simulink model "AccelerationValidation"  (R2022b)
settings: Solver=VariableStepAuto  StartTime=0.0  StopTime=10.0  RelTol=1e-3
(part 1 of 2)
settings Model: Creator=DELL  LastModifiedBy=DELL

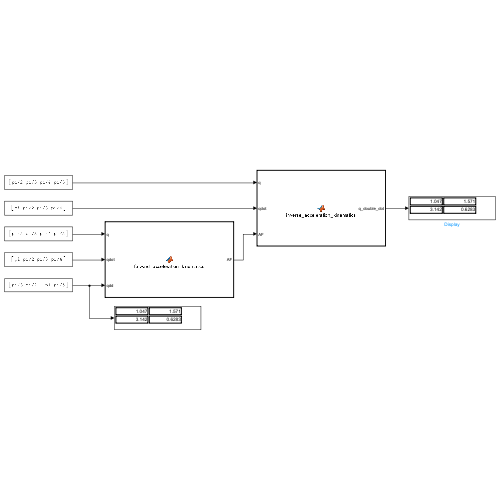
[thumbnail: Simulink's stored preview of the top-level diagram]
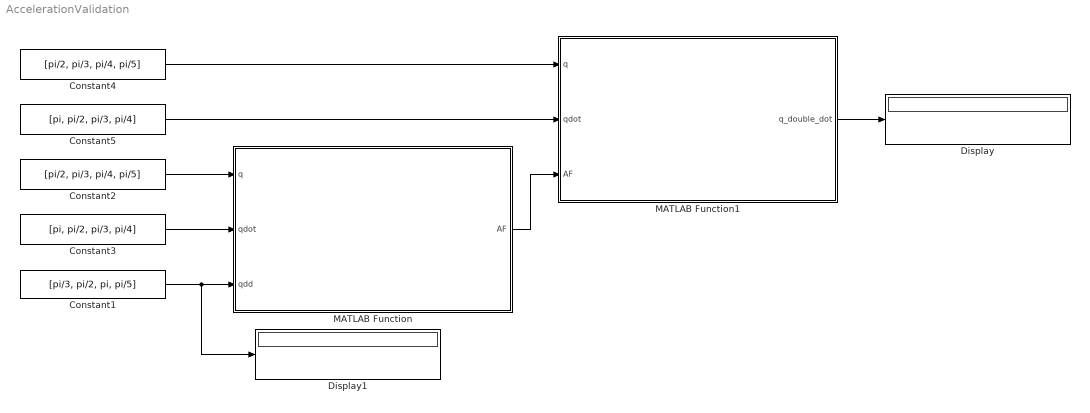
== system AccelerationValidation ==
  Constant1 : Constant  Value=[pi/3, pi/2, pi, pi/5]
  Constant2 : Constant  Value=[pi/2, pi/3, pi/4, pi/5]
  Constant3 : Constant  Value=[pi, pi/2, pi/3, pi/4]
  Constant4 : Constant  Value=[pi/2, pi/3, pi/4, pi/5]
  Constant5 : Constant  Value=[pi, pi/2, pi/3, pi/4]
  Display : Display
  Display1 : Display
  MATLAB Function : MATLAB Function  TreatAsAtomicUnit=on
  MATLAB Function1 : MATLAB Function  TreatAsAtomicUnit=on
  wires:
  Constant2/1 -> MATLAB Function/1(q)
  Constant3/1 -> MATLAB Function/2(qdot)
  Constant1/1 -> Display1/1, MATLAB Function/3(qdd)
  MATLAB Function/1(AF) -> MATLAB Function1/3(AF)
  Constant4/1 -> MATLAB Function1/1(q)
  Constant5/1 -> MATLAB Function1/2(qdot)
  MATLAB Function1/1(q_double_dot) -> Display/1

== matlab function AccelerationValidation/MATLAB Function1 ==
  data: q_double_dot output; q input; qdot input; AF input
function q_double_dot = inverse_acceleration_kinematics(q, qdot, AF)

q1 = q(1);
q2 = q(2);
q3 = q(3);
q4 = q(4);
q1dot = qdot(1);
q2dot = qdot(2);
q3dot = qdot(3);
q4dot = qdot(4);

J =[150*sin(q2)*sin(q1 - pi/2)*sin(q4 - pi/2) - 150*cos(q4 - pi/2)*(cos(q1 - pi/2)*sin(q3 - pi/2) + cos(q2)*cos(q3 - pi/2)*sin(q1 - pi/2)) - 185*sin(q2)*sin(q1 - pi/2),                                                                                                                                                                                                                                                                      -cos(q1 - pi/2)*(150*cos(q2)*sin(q4 - pi/2) - 185*cos(q2) + 150*cos(q3 - pi/2)*cos(q4 - pi/2)*sin(q2)),                                                                                             - cos(q2)*(185*sin(q2)*sin(q1 - pi/2) + 150*cos(q4 - pi/2)*(cos(q1 - pi/2)*sin(q3 - pi/2) + cos(q2)*cos(q3 - pi/2)*sin(q1 - pi/2)) - 150*sin(q2)*sin(q1 - pi/2)*sin(q4 - pi/2)) - sin(q2)*sin(q1 - pi/2)*(150*cos(q2)*sin(q4 - pi/2) - 185*cos(q2) + 150*cos(q3 - pi/2)*cos(q4 - pi/2)*sin(q2)),                                                                                                                - (150*cos(q2)*sin(q4 - pi/2) + 150*cos(q3 - pi/2)*cos(q4 - pi/2)*sin(q2))*(cos(q1 - pi/2)*cos(q3 - pi/2) - cos(q2)*sin(q1 - pi/2)*sin(q3 - pi/2)) - sin(q2)*sin(q3 - pi/2)*(150*cos(q4 - pi/2)*(cos(q1 - pi/2)*sin(q3 - pi/2) + cos(q2)*cos(q3 - pi/2)*sin(q1 - pi/2)) - 150*sin(q2)*sin(q1 - pi/2)*sin(q4 - pi/2));
185*cos(q1 - pi/2)*sin(q2) - 150*cos(q4 - pi/2)*(sin(q1 - pi/2)*sin(q3 - pi/2) - cos(q2)*cos(q1 - pi/2)*cos(q3 - pi/2)) - 150*cos(q1 - pi/2)*sin(q2)*sin(q4 - pi/2),                                                                                                                                                                                                                                                                      -sin(q1 - pi/2)*(150*cos(q2)*sin(q4 - pi/2) - 185*cos(q2) + 150*cos(q3 - pi/2)*cos(q4 - pi/2)*sin(q2)),                                                                                               cos(q1 - pi/2)*sin(q2)*(150*cos(q2)*sin(q4 - pi/2) - 185*cos(q2) + 150*cos(q3 - pi/2)*cos(q4 - pi/2)*sin(q2)) - cos(q2)*(150*cos(q4 - pi/2)*(sin(q1 - pi/2)*sin(q3 - pi/2) - cos(q2)*cos(q1 - pi/2)*cos(q3 - pi/2)) - 185*cos(q1 - pi/2)*sin(q2) + 150*cos(q1 - pi/2)*sin(q2)*sin(q4 - pi/2)),                                                                                                                - (150*cos(q2)*sin(q4 - pi/2) + 150*cos(q3 - pi/2)*cos(q4 - pi/2)*sin(q2))*(cos(q3 - pi/2)*sin(q1 - pi/2) + cos(q2)*cos(q1 - pi/2)*sin(q3 - pi/2)) - sin(q2)*sin(q3 - pi/2)*(150*cos(q4 - pi/2)*(sin(q1 - pi/2)*sin(q3 - pi/2) - cos(q2)*cos(q1 - pi/2)*cos(q3 - pi/2)) + 150*cos(q1 - pi/2)*sin(q2)*sin(q4 - pi/2));
                                                                                                                                                                  0, cos(q1 - pi/2)*(150*cos(q4 - pi/2)*(sin(q1 - pi/2)*sin(q3 - pi/2) - cos(q2)*cos(q1 - pi/2)*cos(q3 - pi/2)) - 185*cos(q1 - pi/2)*sin(q2) + 150*cos(q1 - pi/2)*sin(q2)*sin(q4 - pi/2)) - sin(q1 - pi/2)*(185*sin(q2)*sin(q1 - pi/2) + 150*cos(q4 - pi/2)*(cos(q1 - pi/2)*sin(q3 - pi/2) + cos(q2)*cos(q3 - pi/2)*sin(q1 - pi/2)) - 150*sin(q2)*sin(q1 - pi/2)*sin(q4 - pi/2)), sin(q2)*sin(q1 - pi/2)*(150*cos(q4 - pi/2)*(sin(q1 - pi/2)*sin(q3 - pi/2) - cos(q2)*cos(q1 - pi/2)*cos(q3 - pi/2)) - 185*cos(q1 - pi/2)*sin(q2) + 150*cos(q1 - pi/2)*sin(q2)*sin(q4 - pi/2)) + cos(q1 - pi/2)*sin(q2)*(185*sin(q2)*sin(q1 - pi/2) + 150*cos(q4 - pi/2)*(cos(q1 - pi/2)*sin(q3 - pi/2) + cos(q2)*cos(q3 - pi/2)*sin(q1 - pi/2)) - 150*sin(q2)*sin(q1 - pi/2)*sin(q4 - pi/2)), (150*cos(q4 - pi/2)*(sin(q1 - pi/2)*sin(q3 - pi/2) - cos(q2)*cos(q1 - pi/2)*cos(q3 - pi/2)) + 150*cos(q1 - pi/2)*sin(q2)*sin(q4 - pi/2))*(cos(q1 - pi/2)*cos(q3 - pi/2) - cos(q2)*sin(q1 - pi/2)*sin(q3 - pi/2)) - (150*cos(q4 - pi/2)*(cos(q1 - pi/2)*sin(q3 - pi/2) + cos(q2)*cos(q3 - pi/2)*sin(q1 - pi/2)) - 150*sin(q2)*sin(q1 - pi/2)*sin(q4 - pi/2))*(cos(q3 - pi/2)*sin(q1 - pi/2) + cos(q2)*cos(q1 - pi/2)*sin(q3 - pi/2));
                                                                                                                                                                  0,                                                                                                                                                                                                                                                                                                                                                             -sin(q1 - pi/2),                                                                                                                                                                                                                                                                                                                                                                      cos(q1 - pi/2)*sin(q2),                                                                                                                                                                                                                                                                                                                                                             - cos(q3 - pi/2)*sin(q1 - pi/2) - cos(q2)*cos(q1 - pi/2)*sin(q3 - pi/2);
                                                                                                                                                              0,                                                                                                                                                                                                                                                                                                                                                              cos(q1 - pi/2),                                                                                                                                                                                                                                                                                                                                                                      sin(q2)*sin(q1 - pi/2),                                                                                                                                                                                                                                                                                                                                                               cos(q1 - pi/2)*cos(q3 - pi/2) - cos(q2)*sin(q1 - pi/2)*sin(q3 - pi/2);                                                                                                                                                                  1,                                                                                                                                                                                                                                                                                                                                                                           0,                                                                                                                                                                                                                                                                                                                                                                                     cos(q2),                                                                                                                                                                                                                                                                                                                                                                                                              sin(q2)*sin(q3 - pi/2)];
Jinv = pinv(J);
J_dot = [q4dot*(150*sin(q4 - pi/2)*(cos(q1 - pi/2)*sin(q3 - pi/2) + cos(q2)*cos(q3 - pi/2)*sin(q1 - pi/2)) + 150*cos(q4 - pi/2)*sin(q2)*sin(q1 - pi/2)) + q1dot*(150*cos(q4 - pi/2)*(sin(q1 - pi/2)*sin(q3 - pi/2) - cos(q2)*cos(q1 - pi/2)*cos(q3 - pi/2)) - 185*cos(q1 - pi/2)*sin(q2) + 150*cos(q1 - pi/2)*sin(q2)*sin(q4 - pi/2)) + q2dot*(150*cos(q2)*sin(q1 - pi/2)*sin(q4 - pi/2) - 185*cos(q2)*sin(q1 - pi/2) + 150*cos(q3 - pi/2)*cos(q4 - pi/2)*sin(q2)*sin(q1 - pi/2)) - 150*q3dot*cos(q4 - pi/2)*(cos(q1 - pi/2)*cos(q3 - pi/2) - cos(q2)*sin(q1 - pi/2)*sin(q3 - pi/2)),                                                                                                                                                                                                                                                                                                                                                                                                                                                                                  q1dot*sin(q1 - pi/2)*(150*cos(q2)*sin(q4 - pi/2) - 185*cos(q2) + 150*cos(q3 - pi/2)*cos(q4 - pi/2)*sin(q2)) - q4dot*cos(q1 - pi/2)*(150*cos(q2)*cos(q4 - pi/2) - 150*cos(q3 - pi/2)*sin(q2)*sin(q4 - pi/2)) - q2dot*cos(q1 - pi/2)*(185*sin(q2) - 150*sin(q2)*sin(q4 - pi/2) + 150*cos(q2)*cos(q3 - pi/2)*cos(q4 - pi/2)) + 150*q3dot*cos(q1 - pi/2)*cos(q4 - pi/2)*sin(q2)*sin(q3 - pi/2),        q4dot*(cos(q2)*(150*sin(q4 - pi/2)*(cos(q1 - pi/2)*sin(q3 - pi/2) + cos(q2)*cos(q3 - pi/2)*sin(q1 - pi/2)) + 150*cos(q4 - pi/2)*sin(q2)*sin(q1 - pi/2)) - sin(q2)*sin(q1 - pi/2)*(150*cos(q2)*cos(q4 - pi/2) - 150*cos(q3 - pi/2)*sin(q2)*sin(q4 - pi/2))) - q3dot*(150*cos(q2)*cos(q4 - pi/2)*(cos(q1 - pi/2)*cos(q3 - pi/2) - cos(q2)*sin(q1 - pi/2)*sin(q3 - pi/2)) - 150*cos(q4 - pi/2)*sin(q2)^2*sin(q1 - pi/2)*sin(q3 - pi/2)) + q1dot*(cos(q2)*(150*cos(q4 - pi/2)*(sin(q1 - pi/2)*sin(q3 - pi/2) - cos(q2)*cos(q1 - pi/2)*cos(q3 - pi/2)) - 185*cos(q1 - pi/2)*sin(q2) + 150*cos(q1 - pi/2)*sin(q2)*sin(q4 - pi/2)) - cos(q1 - pi/2)*sin(q2)*(150*cos(q2)*sin(q4 - pi/2) - 185*cos(q2) + 150*cos(q3 - pi/2)*cos(q4 - pi/2)*sin(q2))) + q2dot*(cos(q2)*(150*cos(q2)*sin(q1 - pi/2)*sin(q4 - pi/2) - 185*cos(q2)*sin(q1 - pi/2) + 150*cos(q3 - pi/2)*cos(q4 - pi/2)*sin(q2)*sin(q1 - pi/2)) + sin(q2)*(185*sin(q2)*sin(q1 - pi/2) + 150*cos(q4 - pi/2)*(cos(q1 - pi/2)*sin(q3 - pi/2) + cos(q2)*cos(q3 - pi/2)*sin(q1 - pi/2)) - 150*sin(q2)*sin(q1 - pi/2)*sin(q4 - pi/2)) - sin(q2)*sin(q1 - pi/2)*(185*sin(q2) - 150*sin(q2)*sin(q4 - pi/2) + 150*cos(q2)*cos(q3 - pi/2)*cos(q4 - pi/2)) - cos(q2)*sin(q1 - pi/2)*(150*cos(q2)*sin(q4 - pi/2) - 185*cos(q2) + 150*cos(q3 - pi/2)*cos(q4 - pi/2)*sin(q2))),                                                                    q1dot*((150*cos(q2)*sin(q4 - pi/2) + 150*cos(q3 - pi/2)*cos(q4 - pi/2)*sin(q2))*(cos(q3 - pi/2)*sin(q1 - pi/2) + cos(q2)*cos(q1 - pi/2)*sin(q3 - pi/2)) + sin(q2)*sin(q3 - pi/2)*(150*cos(q4 - pi/2)*(sin(q1 - pi/2)*sin(q3 - pi/2) - cos(q2)*cos(q1 - pi/2)*cos(q3 - pi/2)) + 150*cos(q1 - pi/2)*sin(q2)*sin(q4 - pi/2))) + q3dot*((150*cos(q2)*sin(q4 - pi/2) + 150*cos(q3 - pi/2)*cos(q4 - pi/2)*sin(q2))*(cos(q1 - pi/2)*sin(q3 - pi/2) + cos(q2)*cos(q3 - pi/2)*sin(q1 - pi/2)) - cos(q3 - pi/2)*sin(q2)*(150*cos(q4 - pi/2)*(cos(q1 - pi/2)*sin(q3 - pi/2) + cos(q2)*cos(q3 - pi/2)*sin(q1 - pi/2)) - 150*sin(q2)*sin(q1 - pi/2)*sin(q4 - pi/2))) - q4dot*((150*cos(q2)*cos(q4 - pi/2) - 150*cos(q3 - pi/2)*sin(q2)*sin(q4 - pi/2))*(cos(q1 - pi/2)*cos(q3 - pi/2) - cos(q2)*sin(q1 - pi/2)*sin(q3 - pi/2)) - sin(q2)*sin(q3 - pi/2)*(150*sin(q4 - pi/2)*(cos(q1 - pi/2)*sin(q3 - pi/2) + cos(q2)*cos(q3 - pi/2)*sin(q1 - pi/2)) + 150*cos(q4 - pi/2)*sin(q2)*sin(q1 - pi/2))) + q2dot*((150*sin(q2)*sin(q4 - pi/2) - 150*cos(q2)*cos(q3 - pi/2)*cos(q4 - pi/2))*(cos(q1 - pi/2)*cos(q3 - pi/2) - cos(q2)*sin(q1 - pi/2)*sin(q3 - pi/2)) - cos(q2)*sin(q3 - pi/2)*(150*cos(q4 - pi/2)*(cos(q1 - pi/2)*sin(q3 - pi/2) + cos(q2)*cos(q3 - pi/2)*sin(q1 - pi/2)) - 150*sin(q2)*sin(q1 - pi/2)*sin(q4 - pi/2)) + sin(q2)*sin(q3 - pi/2)*(150*cos(q2)*sin(q1 - pi/2)*sin(q4 - pi/2) + 150*cos(q3 - pi/2)*cos(q4 - pi/2)*sin(q2)*sin(q1 - pi/2)) - sin(q2)*sin(q1 - pi/2)*sin(q3 - pi/2)*(150*cos(q2)*sin(q4 - pi/2) + 150*cos(q3 - pi/2)*cos(q4 - pi/2)*sin(q2)));
q4dot*(150*sin(q4 - pi/2)*(sin(q1 - pi/2)*sin(q3 - pi/2) - cos(q2)*cos(q1 - pi/2)*cos(q3 - pi/2)) - 150*cos(q1 - pi/2)*cos(q4 - pi/2)*sin(q2)) - q2dot*(150*cos(q2)*cos(q1 - pi/2)*sin(q4 - pi/2) - 185*cos(q2)*cos(q1 - pi/2) + 150*cos(q1 - pi/2)*cos(q3 - pi/2)*cos(q4 - pi/2)*sin(q2)) - q1dot*(185*sin(q2)*sin(q1 - pi/2) + 150*cos(q4 - pi/2)*(cos(q1 - pi/2)*sin(q3 - pi/2) + cos(q2)*cos(q3 - pi/2)*sin(q1 - pi/2)) - 150*sin(q2)*sin(q1 - pi/2)*sin(q4 - pi/2)) - 150*q3dot*cos(q4 - pi/2)*(cos(q3 - pi/2)*sin(q1 - pi/2) + cos(q2)*cos(q1 - pi/2)*sin(q3 - pi/2)),                                                                                                                                                                                                                                                                                                                                                                                                                                                                                  150*q3dot*cos(q4 - pi/2)*sin(q2)*sin(q1 - pi/2)*sin(q3 - pi/2) - q1dot*cos(q1 - pi/2)*(150*cos(q2)*sin(q4 - pi/2) - 185*cos(q2) + 150*cos(q3 - pi/2)*cos(q4 - pi/2)*sin(q2)) - q2dot*sin(q1 - pi/2)*(185*sin(q2) - 150*sin(q2)*sin(q4 - pi/2) + 150*cos(q2)*cos(q3 - pi/2)*cos(q4 - pi/2)) - q4dot*sin(q1 - pi/2)*(150*cos(q2)*cos(q4 - pi/2) - 150*cos(q3 - pi/2)*sin(q2)*sin(q4 - pi/2)),        q2dot*(sin(q2)*(150*cos(q4 - pi/2)*(sin(q1 - pi/2)*sin(q3 - pi/2) - cos(q2)*cos(q1 - pi/2)*cos(q3 - pi/2)) - 185*cos(q1 - pi/2)*sin(q2) + 150*cos(q1 - pi/2)*sin(q2)*sin(q4 - pi/2)) - cos(q2)*(150*cos(q2)*cos(q1 - pi/2)*sin(q4 - pi/2) - 185*cos(q2)*cos(q1 - pi/2) + 150*cos(q1 - pi/2)*cos(q3 - pi/2)*cos(q4 - pi/2)*sin(q2)) + cos(q2)*cos(q1 - pi/2)*(150*cos(q2)*sin(q4 - pi/2) - 185*cos(q2) + 150*cos(q3 - pi/2)*cos(q4 - pi/2)*sin(q2)) + cos(q1 - pi/2)*sin(q2)*(185*sin(q2) - 150*sin(q2)*sin(q4 - pi/2) + 150*cos(q2)*cos(q3 - pi/2)*cos(q4 - pi/2))) - q3dot*(150*cos(q2)*cos(q4 - pi/2)*(cos(q3 - pi/2)*sin(q1 - pi/2) + cos(q2)*cos(q1 - pi/2)*sin(q3 - pi/2)) + 150*cos(q1 - pi/2)*cos(q4 - pi/2)*sin(q2)^2*sin(q3 - pi/2)) - q1dot*(cos(q2)*(185*sin(q2)*sin(q1 - pi/2) + 150*cos(q4 - pi/2)*(cos(q1 - pi/2)*sin(q3 - pi/2) + cos(q2)*cos(q3 - pi/2)*sin(q1 - pi/2)) - 150*sin(q2)*sin(q1 - pi/2)*sin(q4 - pi/2)) + sin(q2)*sin(q1 - pi/2)*(150*cos(q2)*sin(q4 - pi/2) - 185*cos(q2) + 150*cos(q3 - pi/2)*cos(q4 - pi/2)*sin(q2))) + q4dot*(cos(q2)*(150*sin(q4 - pi/2)*(sin(q1 - pi/2)*sin(q3 - pi/2) - cos(q2)*cos(q1 - pi/2)*cos(q3 - pi/2)) - 150*cos(q1 - pi/2)*cos(q4 - pi/2)*sin(q2)) + cos(q1 - pi/2)*sin(q2)*(150*cos(q2)*cos(q4 - pi/2) - 150*cos(q3 - pi/2)*sin(q2)*sin(q4 - pi/2))),                                                                    q3dot*((150*cos(q2)*sin(q4 - pi/2) + 150*cos(q3 - pi/2)*cos(q4 - pi/2)*sin(q2))*(sin(q1 - pi/2)*sin(q3 - pi/2) - cos(q2)*cos(q1 - pi/2)*cos(q3 - pi/2)) - cos(q3 - pi/2)*sin(q2)*(150*cos(q4 - pi/2)*(sin(q1 - pi/2)*sin(q3 - pi/2) - cos(q2)*cos(q1 - pi/2)*cos(q3 - pi/2)) + 150*cos(q1 - pi/2)*sin(q2)*sin(q4 - pi/2))) - q4dot*((150*cos(q2)*cos(q4 - pi/2) - 150*cos(q3 - pi/2)*sin(q2)*sin(q4 - pi/2))*(cos(q3 - pi/2)*sin(q1 - pi/2) + cos(q2)*cos(q1 - pi/2)*sin(q3 - pi/2)) - sin(q2)*sin(q3 - pi/2)*(150*sin(q4 - pi/2)*(sin(q1 - pi/2)*sin(q3 - pi/2) - cos(q2)*cos(q1 - pi/2)*cos(q3 - pi/2)) - 150*cos(q1 - pi/2)*cos(q4 - pi/2)*sin(q2))) - q1dot*((150*cos(q2)*sin(q4 - pi/2) + 150*cos(q3 - pi/2)*cos(q4 - pi/2)*sin(q2))*(cos(q1 - pi/2)*cos(q3 - pi/2) - cos(q2)*sin(q1 - pi/2)*sin(q3 - pi/2)) + sin(q2)*sin(q3 - pi/2)*(150*cos(q4 - pi/2)*(cos(q1 - pi/2)*sin(q3 - pi/2) + cos(q2)*cos(q3 - pi/2)*sin(q1 - pi/2)) - 150*sin(q2)*sin(q1 - pi/2)*sin(q4 - pi/2))) + q2dot*((150*sin(q2)*sin(q4 - pi/2) - 150*cos(q2)*cos(q3 - pi/2)*cos(q4 - pi/2))*(cos(q3 - pi/2)*sin(q1 - pi/2) + cos(q2)*cos(q1 - pi/2)*sin(q3 - pi/2)) - cos(q2)*sin(q3 - pi/2)*(150*cos(q4 - pi/2)*(sin(q1 - pi/2)*sin(q3 - pi/2) - cos(q2)*cos(q1 - pi/2)*cos(q3 - pi/2)) + 150*cos(q1 - pi/2)*sin(q2)*sin(q4 - pi/2)) - sin(q2)*sin(q3 - pi/2)*(150*cos(q2)*cos(q1 - pi/2)*sin(q4 - pi/2) + 150*cos(q1 - pi/2)*cos(q3 - pi/2)*cos(q4 - pi/2)*sin(q2)) + cos(q1 - pi/2)*sin(q2)*sin(q3 - pi/2)*(150*cos(q2)*sin(q4 - pi/2) + 150*cos(q3 - pi/2)*cos(q4 - pi/2)*sin(q2)));
                                                                                                                                                                                                                                                                                                                                                                                                                                                                                                                                                                          0, q3dot*(150*cos(q1 - pi/2)*cos(q4 - pi/2)*(cos(q3 - pi/2)*sin(q1 - pi/2) + cos(q2)*cos(q1 - pi/2)*sin(q3 - pi/2)) - 150*cos(q4 - pi/2)*sin(q1 - pi/2)*(cos(q1 - pi/2)*cos(q3 - pi/2) - cos(q2)*sin(q1 - pi/2)*sin(q3 - pi/2))) - q4dot*(cos(q1 - pi/2)*(150*sin(q4 - pi/2)*(sin(q1 - pi/2)*sin(q3 - pi/2) - cos(q2)*cos(q1 - pi/2)*cos(q3 - pi/2)) - 150*cos(q1 - pi/2)*cos(q4 - pi/2)*sin(q2)) - sin(q1 - pi/2)*(150*sin(q4 - pi/2)*(cos(q1 - pi/2)*sin(q3 - pi/2) + cos(q2)*cos(q3 - pi/2)*sin(q1 - pi/2)) + 150*cos(q4 - pi/2)*sin(q2)*sin(q1 - pi/2))) + q2dot*(cos(q1 - pi/2)*(150*cos(q2)*cos(q1 - pi/2)*sin(q4 - pi/2) - 185*cos(q2)*cos(q1 - pi/2) + 150*cos(q1 - pi/2)*cos(q3 - pi/2)*cos(q4 - pi/2)*sin(q2)) + sin(q1 - pi/2)*(150*cos(q2)*sin(q1 - pi/2)*sin(q4 - pi/2) - 185*cos(q2)*sin(q1 - pi/2) + 150*cos(q3 - pi/2)*cos(q4 - pi/2)*sin(q2)*sin(q1 - pi/2))), q2dot*(sin(q2)*sin(q1 - pi/2)*(150*cos(q2)*cos(q1 - pi/2)*sin(q4 - pi/2) - 185*cos(q2)*cos(q1 - pi/2) + 150*cos(q1 - pi/2)*cos(q3 - pi/2)*cos(q4 - pi/2)*sin(q2)) + cos(q2)*sin(q1 - pi/2)*(150*cos(q4 - pi/2)*(sin(q1 - pi/2)*sin(q3 - pi/2) - cos(q2)*cos(q1 - pi/2)*cos(q3 - pi/2)) - 185*cos(q1 - pi/2)*sin(q2) + 150*cos(q1 - pi/2)*sin(q2)*sin(q4 - pi/2)) + cos(q2)*cos(q1 - pi/2)*(185*sin(q2)*sin(q1 - pi/2) + 150*cos(q4 - pi/2)*(cos(q1 - pi/2)*sin(q3 - pi/2) + cos(q2)*cos(q3 - pi/2)*sin(q1 - pi/2)) - 150*sin(q2)*sin(q1 - pi/2)*sin(q4 - pi/2)) - cos(q1 - pi/2)*sin(q2)*(150*cos(q2)*sin(q1 - pi/2)*sin(q4 - pi/2) - 185*cos(q2)*sin(q1 - pi/2) + 150*cos(q3 - pi/2)*cos(q4 - pi/2)*sin(q2)*sin(q1 - pi/2))) - q4dot*(cos(q1 - pi/2)*sin(q2)*(150*sin(q4 - pi/2)*(cos(q1 - pi/2)*sin(q3 - pi/2) + cos(q2)*cos(q3 - pi/2)*sin(q1 - pi/2)) + 150*cos(q4 - pi/2)*sin(q2)*sin(q1 - pi/2)) + sin(q2)*sin(q1 - pi/2)*(150*sin(q4 - pi/2)*(sin(q1 - pi/2)*sin(q3 - pi/2) - cos(q2)*cos(q1 - pi/2)*cos(q3 - pi/2)) - 150*cos(q1 - pi/2)*cos(q4 - pi/2)*sin(q2))) + q3dot*(150*cos(q1 - pi/2)*cos(q4 - pi/2)*sin(q2)*(cos(q1 - pi/2)*cos(q3 - pi/2) - cos(q2)*sin(q1 - pi/2)*sin(q3 - pi/2)) + 150*cos(q4 - pi/2)*sin(q2)*sin(q1 - pi/2)*(cos(q3 - pi/2)*sin(q1 - pi/2) + cos(q2)*cos(q1 - pi/2)*sin(q3 - pi/2))), q2dot*((150*cos(q2)*cos(q1 - pi/2)*sin(q4 - pi/2) + 150*cos(q1 - pi/2)*cos(q3 - pi/2)*cos(q4 - pi/2)*sin(q2))*(cos(q1 - pi/2)*cos(q3 - pi/2) - cos(q2)*sin(q1 - pi/2)*sin(q3 - pi/2)) + (150*cos(q2)*sin(q1 - pi/2)*sin(q4 - pi/2) + 150*cos(q3 - pi/2)*cos(q4 - pi/2)*sin(q2)*sin(q1 - pi/2))*(cos(q3 - pi/2)*sin(q1 - pi/2) + cos(q2)*cos(q1 - pi/2)*sin(q3 - pi/2)) + cos(q1 - pi/2)*sin(q2)*sin(q3 - pi/2)*(150*cos(q4 - pi/2)*(cos(q1 - pi/2)*sin(q3 - pi/2) + cos(q2)*cos(q3 - pi/2)*sin(q1 - pi/2)) - 150*sin(q2)*sin(q1 - pi/2)*sin(q4 - pi/2)) + sin(q2)*sin(q1 - pi/2)*sin(q3 - pi/2)*(150*cos(q4 - pi/2)*(sin(q1 - pi/2)*sin(q3 - pi/2) - cos(q2)*cos(q1 - pi/2)*cos(q3 - pi/2)) + 150*cos(q1 - pi/2)*sin(q2)*sin(q4 - pi/2))) - q3dot*((150*cos(q4 - pi/2)*(sin(q1 - pi/2)*sin(q3 - pi/2) - cos(q2)*cos(q1 - pi/2)*cos(q3 - pi/2)) + 150*cos(q1 - pi/2)*sin(q2)*sin(q4 - pi/2))*(cos(q1 - pi/2)*sin(q3 - pi/2) + cos(q2)*cos(q3 - pi/2)*sin(q1 - pi/2)) - (150*cos(q4 - pi/2)*(cos(q1 - pi/2)*sin(q3 - pi/2) + cos(q2)*cos(q3 - pi/2)*sin(q1 - pi/2)) - 150*sin(q2)*sin(q1 - pi/2)*sin(q4 - pi/2))*(sin(q1 - pi/2)*sin(q3 - pi/2) - cos(q2)*cos(q1 - pi/2)*cos(q3 - pi/2))) - q4dot*((150*sin(q4 - pi/2)*(sin(q1 - pi/2)*sin(q3 - pi/2) - cos(q2)*cos(q1 - pi/2)*cos(q3 - pi/2)) - 150*cos(q1 - pi/2)*cos(q4 - pi/2)*sin(q2))*(cos(q1 - pi/2)*cos(q3 - pi/2) - cos(q2)*sin(q1 - pi/2)*sin(q3 - pi/2)) - (150*sin(q4 - pi/2)*(cos(q1 - pi/2)*sin(q3 - pi/2) + cos(q2)*cos(q3 - pi/2)*sin(q1 - pi/2)) + 150*cos(q4 - pi/2)*sin(q2)*sin(q1 - pi/2))*(cos(q3 - pi/2)*sin(q1 - pi/2) + cos(q2)*cos(q1 - pi/2)*sin(q3 - pi/2)));
                                                                                                                                                                                                                                                                                                                                                                                                                                                                                                                                                                          0,                                                                                                                                                                                                                                                                                                                                                                                                                                                                                                                                                                                                                                                                                                                                                                                                                                                       -q1dot*cos(q1 - pi/2),                                                                                                                                                                                                                                                                                                                                                                                                                                                                                                                                                                                                                                                                                                                                                                                                                                                                                                                                                                                                                                                                                                                                                                                                                                                               q2dot*cos(q2)*cos(q1 - pi/2) - q1dot*sin(q2)*sin(q1 - pi/2),                                                                                                                                                                                                                                                                                                                                                                                                                                                                                                                                                                                                                                                                                                                                                                                                                                                                                                                                                                                                                                                                                                                                                                                                                                                                                                                                                                                                                           q3dot*(sin(q1 - pi/2)*sin(q3 - pi/2) - cos(q2)*cos(q1 - pi/2)*cos(q3 - pi/2)) - q1dot*(cos(q1 - pi/2)*cos(q3 - pi/2) - cos(q2)*sin(q1 - pi/2)*sin(q3 - pi/2)) + q2dot*cos(q1 - pi/2)*sin(q2)*sin(q3 - pi/2);
                                                                                                                                                                                                                                                                                                                                                                                                                                                                                                                                                                          0,                                                                                                                                                                                                                                                                                                                                                                                                                                                                                                                                                                                                                                                                                                                                                                                                                                                       -q1dot*sin(q1 - pi/2),                                                                                                                                                                                                                                                                                                                                                                                                                                                                                                                                                                                                                                                                                                                                                                                                                                                                                                                                                                                                                                                                                                                                                                                                                                                               q1dot*cos(q1 - pi/2)*sin(q2) + q2dot*cos(q2)*sin(q1 - pi/2),                                                                                                                                                                                                                                                                                                                                                                                                                                                                                                                                                                                                                                                                                                                                                                                                                                                                                                                                                                                                                                                                                                                                                                                                                                                                                                                                                                                                                           q2dot*sin(q2)*sin(q1 - pi/2)*sin(q3 - pi/2) - q3dot*(cos(q1 - pi/2)*sin(q3 - pi/2) + cos(q2)*cos(q3 - pi/2)*sin(q1 - pi/2)) - q1dot*(cos(q3 - pi/2)*sin(q1 - pi/2) + cos(q2)*cos(q1 - pi/2)*sin(q3 - pi/2));
                                                                                                                                                                                                                                                                                                                                                                                                                                                                                                                                                                          0,                                                                                                                                                                                                                                                                                                                                                                                                                                                                                                                                                                                                                                                                                                                                                                                                                                                                           0,                                                                                                                                                                                                                                                                                                                                                                                                                                                                                                                                                                                                                                                                                                                                                                                                                                                                                                                                                                                                                                                                                                                                                                                                                                                                                                            -q2dot*sin(q2),                                                                                                                                                                                                                                                                                                                                                                                                                                                                                                                                                                                                                                                                                                                                                                                                                                                                                                                                                                                                                                                                                                                                                                                                                                                                                                                                                                                                                                                                                                                                                                           q2dot*cos(q2)*sin(q3 - pi/2) + q3dot*cos(q3 - pi/2)*sin(q2)];
 
q_double_dot = Jinv * (AF - J_dot * [q1dot; q2dot; q3dot; q4dot]);

end
